simulink model "sampleModel1495_3"  (R2023a)
settings: Solver=VariableStepAuto  StartTime=0.0  StopTime=10.0  RelTol=1e-3
libraries: hdlsllib x6
settings Model: Creator=user1  LastModifiedBy=user1

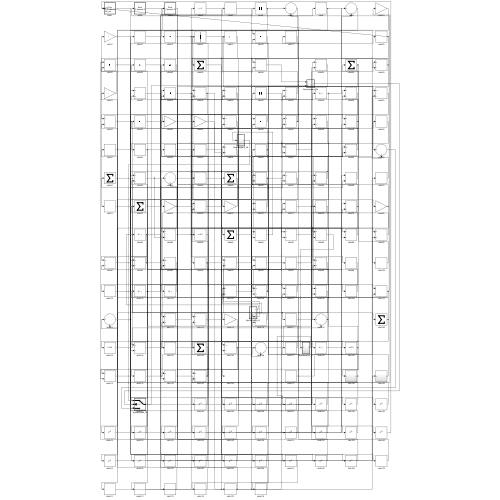
[thumbnail: Simulink's stored preview of the top-level diagram]
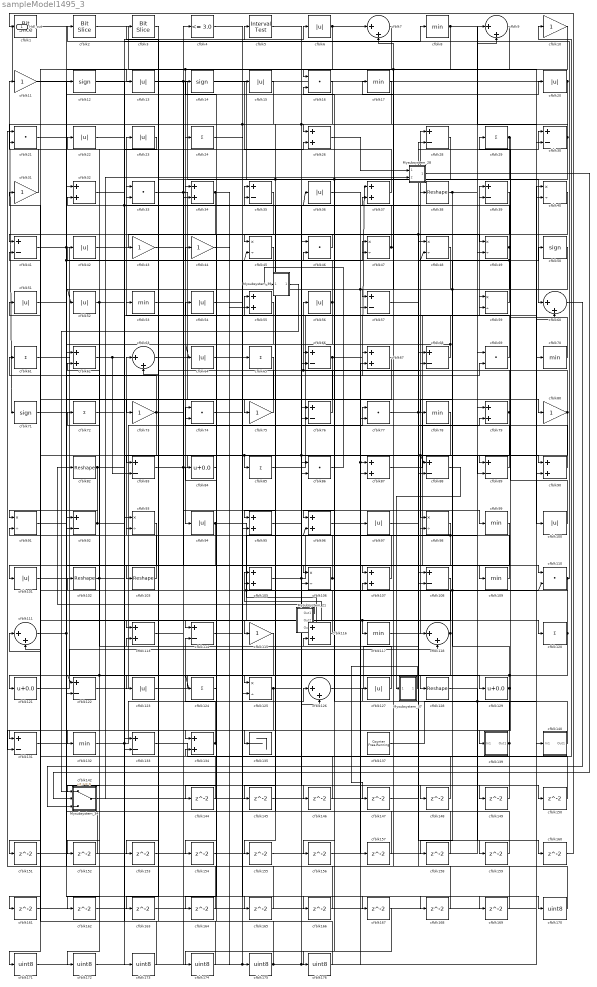
== system sampleModel1495_3 ==
  Mysubsystem_21 : Subsystem  TreatAsAtomicUnit=on  RTWFcnName=Mysubsystem_21
      settings: RTWFcnNameOpts=User specified  RTWFileNameOpts=Use function name
  Mysubsystem_28 : Subsystem  TreatAsAtomicUnit=on  RTWFcnName=Mysubsystem_28
      settings: RTWFcnNameOpts=User specified  RTWFileNameOpts=Use function name
  Mysubsystem_34 : Subsystem  TreatAsAtomicUnit=on  RTWFcnName=Mysubsystem_34
      settings: RTWFcnNameOpts=User specified  RTWFileNameOpts=Use function name
  Mysubsystem_37 : Subsystem  TreatAsAtomicUnit=on  RTWFcnName=Mysubsystem_37
      settings: RTWFcnNameOpts=User specified  RTWFileNameOpts=Use function name
  Mysubsystem_39 : Subsystem  TreatAsAtomicUnit=on  RTWFcnName=Mysubsystem_39
      settings: RTWFcnNameOpts=User specified  RTWFileNameOpts=Use function name
  cfblk1 : hdlsllib/Logic and Bit Operations/Bit Slice  lidx=7  ridx=0
  cfblk{10..11,31,43..44,73,75,80,115} (9 alike) : Gain  OutDataTypeStr=uint8
  cfblk{6,13,15,20,22..23,36,42,51..52,54,56,64,94,97,100..101,123,127} (19 alike) : Abs  OutDataTypeStr=uint8  SaturateOnIntegerOverflow=off
  cfblk{38,82,102..103,128} (5 alike) : Reshape
  cfblk{26,32,34,37,55,62,67,79,87,90,95..96,105,107,113,116,134} (17 alike) : Sum  OutDataTypeStr=uint8
  cfblk{40,45,47..49,59,91,93,98,106,125} (11 alike) : Product  Inputs=*/  OutDataTypeStr=uint8  RndMeth=Zero  SaturateOnIntegerOverflow=on
  cfblk{28,30,35,39,41,57,66,68,76,83,88..89,92,108,114,122,131,133} (18 alike) : Sum  Inputs=+-  OutDataTypeStr=uint8
  cfblk{8,17,53,70,78,99,109,117,132} (9 alike) : MinMax  OutDataTypeStr=uint8
  cfblk{16,21,33,46,69,74,77,86,110} (9 alike) : DotProduct  OutDataTypeStr=uint8
  cfblk{7,9,60,63,111,118,126} (7 alike) : Sum  Inputs=|++  OutDataTypeStr=uint8
  cfblk{12,14,50,71} (4 alike) : Signum
  cfblk{24,29,61,65,72,85,120,124} (8 alike) : Sum  Inputs=+  OutDataTypeStr=uint8
  cfblk121 : Bias  Bias=0.0  SaturateOnIntegerOverflow=off
  cfblk129 : Bias  Bias=0.0  SaturateOnIntegerOverflow=off
  cfblk135 : Terminator
  cfblk137 : hdlsllib/Sources/Counter Free-Running  NumBits=16  tsamp=-1
  cfblk139 : Subsystem
      settings: LibrarySourceBlock=|
      | hdlsllib/Ports &
      | Subsystems/Subsystem
  cfblk140 : Subsystem
      settings: LibrarySourceBlock=|
      | hdlsllib/Ports &
      | Subsystems/Subsystem
  cfblk142 : Switch  OutDataTypeStr=uint8  SaturateOnIntegerOverflow=off  InputSameDT=off
  cfblk{144..169} (26 alike) : Delay  SampleTime=1
  cfblk{170..176} (7 alike) : DataTypeConversion  OutDataTypeStr=uint8  SaturateOnIntegerOverflow=off  RndMeth=Floor
  cfblk2 : hdlsllib/Logic and Bit Operations/Bit Slice  lidx=7  ridx=0
  cfblk3 : hdlsllib/Logic and Bit Operations/Bit Slice  lidx=7  ridx=0
  cfblk4 : hdlsllib/Logic and Bit Operations/Compare To Constant  relop=<=  const=3.0  OutDataTypeStr=uint8
  cfblk5 : hdlsllib/Logic and Bit Operations/Interval Test  IntervalClosedRight=on  uplimit=0.5  IntervalClosedLeft=on  lowlimit=-0.5  OutDataTypeStr=uint8
  cfblk84 : Bias  Bias=0.0  SaturateOnIntegerOverflow=off
  Hdl_out : Outport  OutDataTypeStr=uint8
  wires:
  cfblk41/1 -> cfblk45/2, cfblk165/1, cfblk129/1
  cfblk16/1 -> cfblk71/1, cfblk125/2
  cfblk63/1 -> cfblk80/1
  cfblk79/1 -> cfblk56/1, cfblk55/1, cfblk116/1
  cfblk103/1 -> cfblk63/1
  cfblk31/1 -> cfblk11/1
  cfblk117/1 -> cfblk28/1
  cfblk61/1 -> cfblk115/1
  cfblk122/1 -> cfblk77/1
  cfblk110/1 -> cfblk2/1, cfblk105/2
  cfblk20/1 -> cfblk66/2, cfblk145/1, Hdl_out/1
  cfblk132/1 -> cfblk26/2, cfblk36/1, cfblk126/1
  cfblk65/1 -> cfblk101/1
  cfblk17/1 -> cfblk94/1
  cfblk71/1 -> cfblk120/1
  cfblk85/1 -> cfblk39/1
  cfblk93/1 -> cfblk172/1
  cfblk39/1 -> cfblk114/1, cfblk88/2
  cfblk38/1 -> cfblk9/2, cfblk158/1
  cfblk62/1 -> cfblk8/1, cfblk83/2
  cfblk77/1 -> cfblk110/1, cfblk159/1
  cfblk113/1 -> cfblk35/1
  cfblk33/1 -> cfblk75/1, cfblk99/1
  cfblk14/1 -> cfblk100/1
  cfblk9/1 -> cfblk16/1
  cfblk7/1 -> cfblk73/1
  cfblk29/1 -> cfblk139/1(In1), cfblk176/1
  cfblk8/1 -> cfblk34/1, cfblk142/3, cfblk30/2
  cfblk1/1 -> cfblk13/1
  cfblk78/1 -> cfblk98/1, cfblk162/1
  cfblk13/1 -> cfblk60/1, cfblk87/2
  cfblk74/1 -> cfblk46/2
  cfblk94/1 -> cfblk126/2, cfblk171/1
  cfblk45/1 -> cfblk83/1
  cfblk37/1 -> cfblk15/1
  cfblk87/1 -> cfblk40/1
  cfblk70/1 -> cfblk29/1
  cfblk127/1 -> cfblk22/1
  cfblk43/1 -> cfblk49/1
  cfblk69/1 -> cfblk23/1
  cfblk21/1 -> cfblk76/2
  cfblk76/1 -> cfblk32/2
  cfblk137/1 -> cfblk79/1, cfblk70/1
  cfblk120/1 -> cfblk33/1, cfblk98/2, cfblk155/1
  cfblk22/1 -> cfblk86/2
  cfblk111/1 -> cfblk20/1, cfblk167/1
  cfblk36/1 -> cfblk97/1
  cfblk134/1 -> cfblk114/2, cfblk84/1
  cfblk44/1 -> cfblk175/1
  cfblk5/1 -> cfblk89/2, cfblk150/1
  cfblk98/1 -> cfblk96/2, cfblk156/1
  cfblk55/1 -> cfblk123/1
  cfblk56/1 -> cfblk14/1, cfblk142/2
  cfblk82/1 -> cfblk133/1, cfblk122/2
  cfblk52/1 -> cfblk142/1, cfblk5/1
  cfblk106/1 -> cfblk16/2, cfblk31/1
  cfblk6/1 -> cfblk121/1, cfblk7/1
  cfblk34/1 -> cfblk103/1, cfblk55/2
  cfblk109/1 -> cfblk72/1
  cfblk116/1 -> cfblk102/1
  cfblk2/1 -> cfblk60/2
  cfblk102/1 -> cfblk122/1, cfblk152/1, cfblk59/2
  cfblk75/1 -> cfblk3/1
  cfblk72/1 -> cfblk6/1
  cfblk51/1 -> cfblk12/1
  cfblk35/1 -> cfblk92/2
  cfblk42/1 -> cfblk45/1
  cfblk90/1 -> cfblk74/1
  cfblk133/1 -> cfblk10/1
  cfblk108/1 -> cfblk117/1, cfblk131/1
  cfblk24/1 -> cfblk90/1
  cfblk50/1 -> cfblk96/1, cfblk78/1
  cfblk47/1 -> cfblk17/1, cfblk33/2
  cfblk101/1 -> cfblk109/1
  cfblk15/1 -> cfblk24/1
  cfblk142/1 -> cfblk48/1
  cfblk99/1 -> cfblk134/1
  cfblk59/1 -> cfblk42/1
  cfblk139/1(Out1) -> cfblk134/2, cfblk116/2
  cfblk73/1 -> cfblk47/1, cfblk61/1, cfblk151/1
  cfblk140/1(Out1) -> cfblk66/1
  cfblk57/1 -> cfblk50/1
  cfblk92/1 -> cfblk91/1, cfblk69/2
  cfblk66/1 -> cfblk37/1, cfblk132/1
  cfblk129/1 -> cfblk43/1, cfblk124/1, cfblk163/1
  cfblk30/1 -> cfblk106/1, cfblk106/2, cfblk26/1
  cfblk28/1 -> cfblk135/1, cfblk113/1
  cfblk83/1 -> cfblk85/1, cfblk88/1, cfblk89/1
  cfblk125/1 -> cfblk59/1, cfblk131/2
  cfblk123/1 -> cfblk128/1
  cfblk40/1 -> cfblk95/1
  cfblk89/1 -> cfblk54/1
  cfblk100/1 -> cfblk39/2
  cfblk91/1 -> cfblk67/1
  cfblk105/1 -> cfblk9/1, cfblk38/1
  cfblk49/1 -> cfblk52/1, cfblk57/2, cfblk48/2, cfblk7/2
  cfblk95/1 -> cfblk68/2
  cfblk126/1 -> cfblk79/2
  cfblk80/1 -> cfblk108/2, cfblk47/2
  cfblk23/1 -> cfblk21/2
  cfblk107/1 -> cfblk62/2
  cfblk10/1 -> cfblk111/2, cfblk57/1
  cfblk97/1 -> cfblk30/1
  cfblk118/1 -> cfblk133/2, cfblk51/1
  cfblk68/1 -> cfblk53/1, cfblk64/1
  cfblk53/1 -> cfblk107/1
  cfblk121/1 -> cfblk118/2
  cfblk46/1 -> cfblk41/1
  cfblk48/1 -> cfblk125/1
  cfblk67/1 -> cfblk144/1
  cfblk144/1 -> cfblk91/2
  cfblk145/1 -> cfblk28/2
  cfblk114/1 -> cfblk146/1
  cfblk146/1 -> cfblk76/1
  cfblk147/1 -> cfblk108/1
  cfblk54/1 -> cfblk148/1
  cfblk148/1 -> cfblk74/2
  cfblk131/1 -> cfblk149/1
  cfblk149/1 -> cfblk37/2
  cfblk150/1 -> cfblk111/1
  cfblk151/1 -> cfblk34/2
  cfblk152/1 -> cfblk62/1
  cfblk3/1 -> cfblk153/1
  cfblk153/1 -> cfblk49/2
  cfblk84/1 -> cfblk154/1
  cfblk154/1 -> cfblk46/1
  cfblk155/1 -> cfblk69/1
  cfblk156/1 -> cfblk118/1
  cfblk96/1 -> cfblk157/1
  cfblk157/1 -> cfblk35/2
  cfblk158/1 -> cfblk32/1
  cfblk159/1 -> cfblk107/2
  cfblk128/1 -> cfblk160/1
  cfblk160/1 -> cfblk1/1
  cfblk115/1 -> cfblk161/1
  cfblk161/1 -> cfblk40/2
  cfblk162/1 -> cfblk90/2
  cfblk163/1 -> cfblk95/2
  cfblk124/1 -> cfblk164/1
  cfblk164/1 -> cfblk63/2
  cfblk165/1 -> cfblk113/2
  cfblk11/1 -> cfblk166/1
  cfblk166/1 -> cfblk92/1
  cfblk12/1 -> cfblk168/1
  cfblk168/1 -> cfblk21/1
  cfblk64/1 -> cfblk169/1
  cfblk169/1 -> cfblk68/1
  cfblk4/1 -> cfblk170/1
  cfblk170/1 -> cfblk127/1
  cfblk171/1 -> cfblk4/1
  cfblk172/1 -> cfblk140/1(In1), cfblk86/1, cfblk65/1
  cfblk32/1 -> cfblk173/1
  cfblk173/1 -> cfblk93/1
  cfblk167/1 -> cfblk174/1
  cfblk174/1 -> cfblk93/2
  cfblk175/1 -> cfblk87/1, cfblk77/2, cfblk41/2
  cfblk176/1 -> cfblk44/1
  Mysubsystem_21/3(Out3) -> cfblk67/2, cfblk110/2
  Mysubsystem_21/1(Out1) -> cfblk82/1
  Mysubsystem_21/2(Out2) -> cfblk105/1
  cfblk26/1 -> Mysubsystem_28/1(In1)
  Mysubsystem_28/1(Out1) -> Mysubsystem_34/2(In2)
  cfblk60/1 -> Mysubsystem_34/3(In3)
  Mysubsystem_34/1(Out1) -> Mysubsystem_28/2(In2)
  cfblk88/1 -> Mysubsystem_37/1(In1)
  Mysubsystem_37/1(Out1) -> cfblk147/1
  cfblk86/1 -> Mysubsystem_39/1(In1)
  Mysubsystem_39/1(Out1) -> Mysubsystem_34/1(In1)

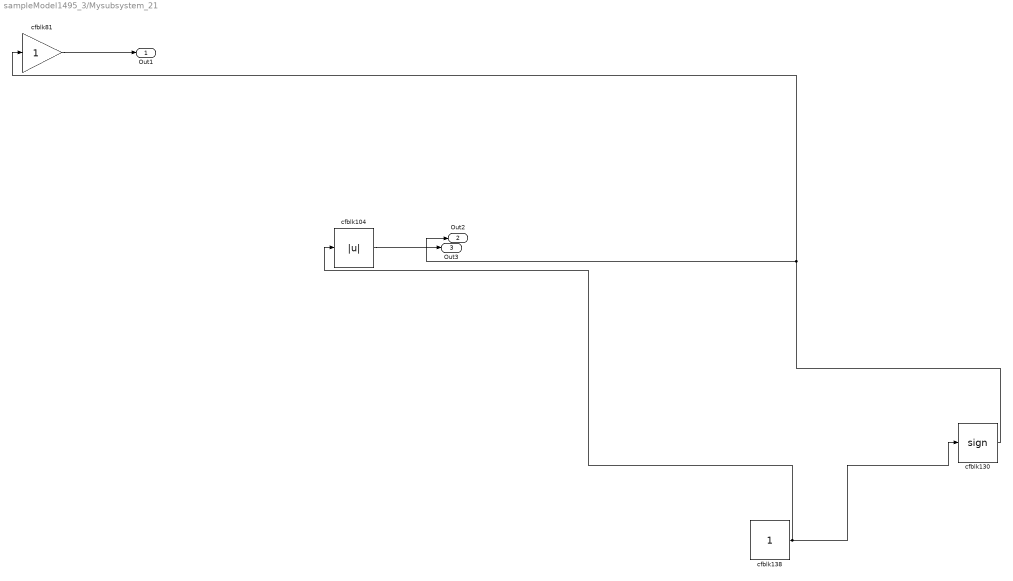
== system sampleModel1495_3/Mysubsystem_21 ==
  cfblk104 : Abs  SaturateOnIntegerOverflow=off
  cfblk130 : Signum
  cfblk138 : Constant  SampleTime=-1
  cfblk81 : Gain
  Out1 : Outport
  Out2 : Outport  Port=2
  Out3 : Outport  Port=3
  wires:
  cfblk138/1 -> cfblk104/1, cfblk130/1
  cfblk130/1 -> Out2/1, cfblk81/1
  cfblk104/1 -> Out3/1
  cfblk81/1 -> Out1/1

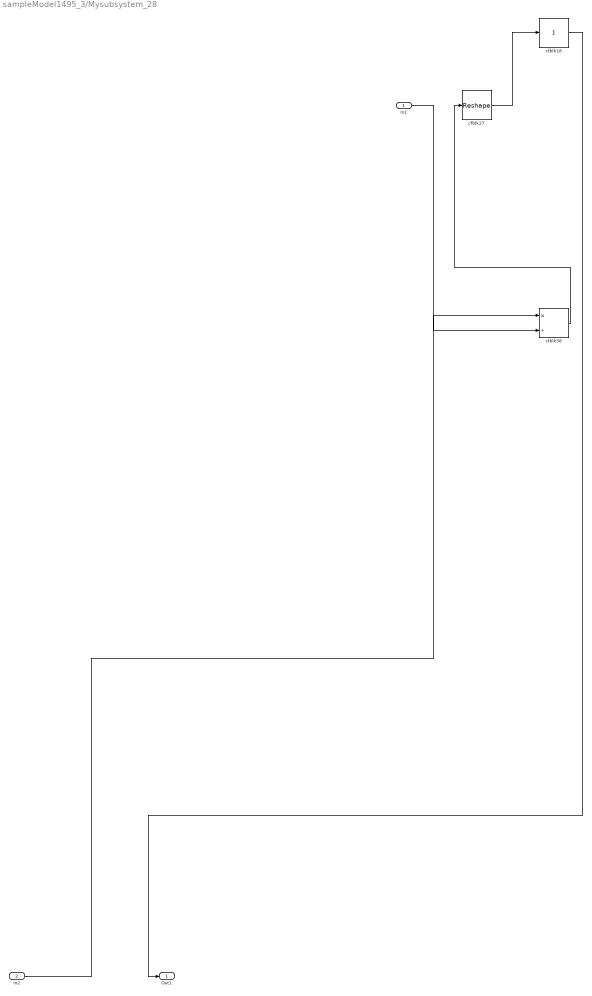
== system sampleModel1495_3/Mysubsystem_28 ==
  In1 : Inport
  In2 : Inport  Port=2
  cfblk18 : Sum  Inputs=+
  cfblk27 : Reshape
  cfblk58 : Product  Inputs=*/  RndMeth=Zero  SaturateOnIntegerOverflow=on
  Out1 : Outport
  wires:
  cfblk18/1 -> Out1/1
  cfblk27/1 -> cfblk18/1
  cfblk58/1 -> cfblk27/1
  In1/1 -> cfblk58/2
  In2/1 -> cfblk58/1

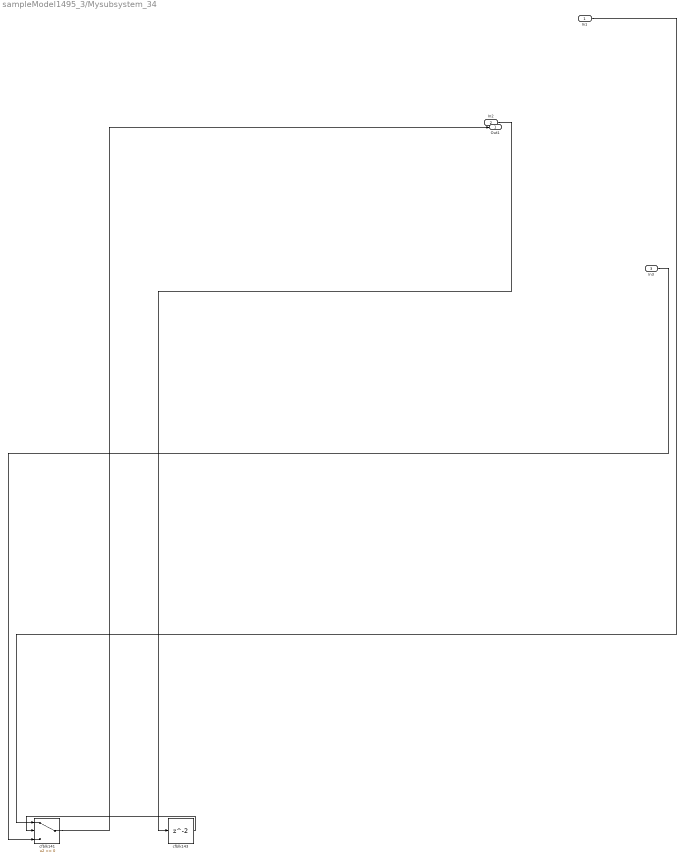
== system sampleModel1495_3/Mysubsystem_34 ==
  In1 : Inport
  In2 : Inport  Port=2
  In3 : Inport  Port=3
  cfblk141 : Switch  SaturateOnIntegerOverflow=off  InputSameDT=off
  cfblk143 : Delay  SampleTime=1
  Out1 : Outport
  wires:
  In1/1 -> cfblk141/1
  cfblk143/1 -> cfblk141/2
  cfblk141/1 -> Out1/1
  In2/1 -> cfblk143/1
  In3/1 -> cfblk141/3

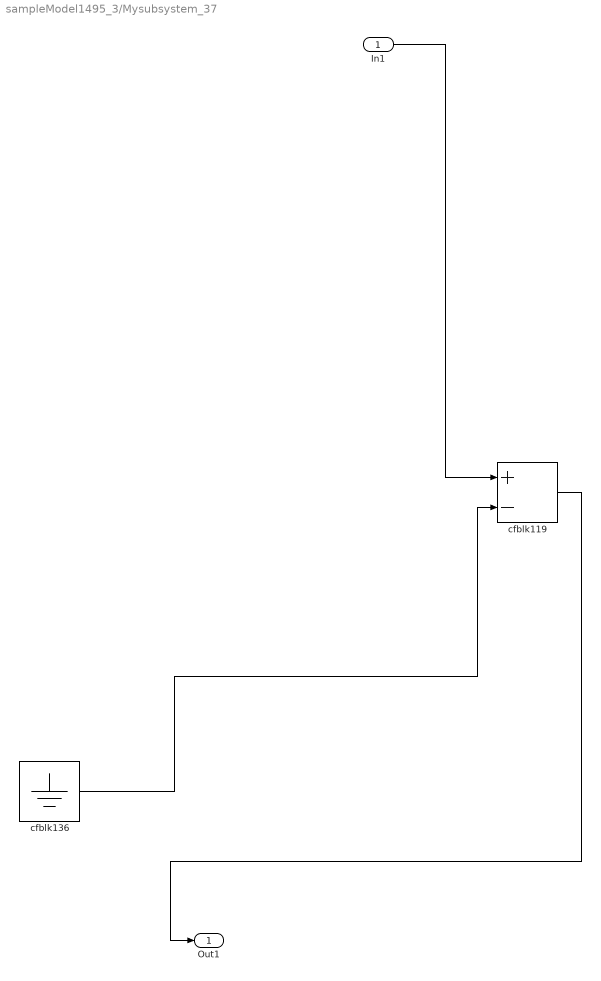
== system sampleModel1495_3/Mysubsystem_37 ==
  In1 : Inport
  cfblk119 : Sum  Inputs=+-
  cfblk136 : Ground
  Out1 : Outport
  wires:
  In1/1 -> cfblk119/1
  cfblk136/1 -> cfblk119/2
  cfblk119/1 -> Out1/1

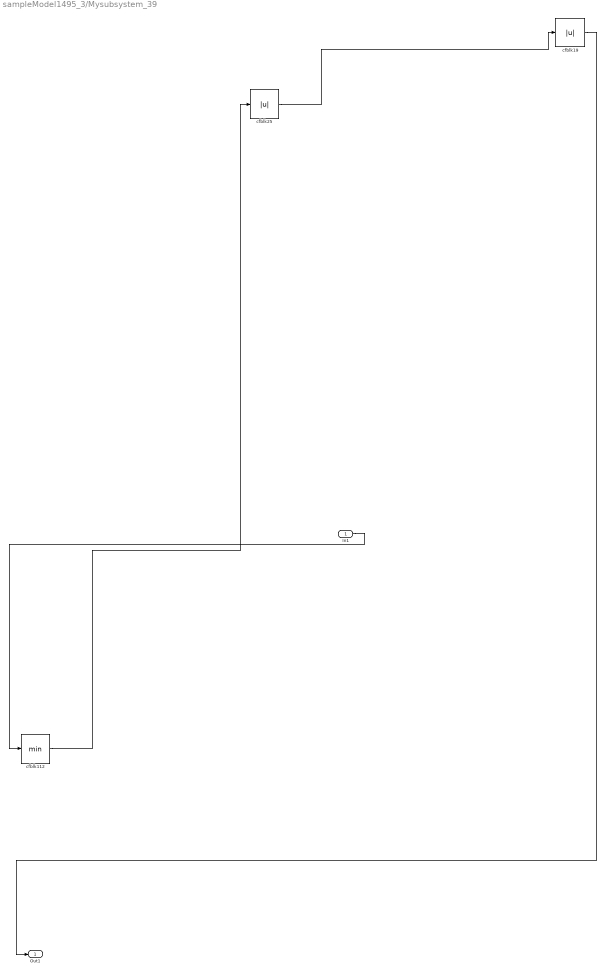
== system sampleModel1495_3/Mysubsystem_39 ==
  In1 : Inport
  cfblk112 : MinMax
  cfblk19 : Abs  SaturateOnIntegerOverflow=off
  cfblk25 : Abs  SaturateOnIntegerOverflow=off
  Out1 : Outport
  wires:
  cfblk112/1 -> cfblk25/1
  cfblk25/1 -> cfblk19/1
  cfblk19/1 -> Out1/1
  In1/1 -> cfblk112/1

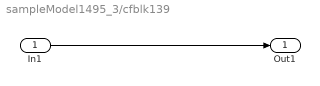
== system sampleModel1495_3/cfblk139 ==
  In1 : Inport
  Out1 : Outport
  wires:
  In1/1 -> Out1/1

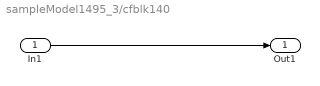
== system sampleModel1495_3/cfblk140 ==
  In1 : Inport
  Out1 : Outport
  wires:
  In1/1 -> Out1/1
